simulink model "asbhl20_FDIRApp1"  (R2013a)
settings: Solver=FixedStepDiscrete  SolverMode=SingleTasking  StartTime=0.0  StopTime=10.0  FixedStep=1/60  RelTol=1e-3
PreLoadFcn:
  | load asbhl20GlobalChildrenData.mat
  | load asbhl20_FDIRAppData.mat
undefined symbols (not defined in the file): Tc, Tf
libraries: asbhl20screen x21, asbhl20_mode_logic x1
Description:
  | HL-20 actuators: fault detection, isolation, and recovery (FDIR) example module
settings Model: FPTRunName=Active  ExtModeAutoUpdateStatusClock=off  BufferReuse=off  Creator=The MathWorks Inc.
settings DataIOCC: LimitDataPoints=off  SaveOutput=off  SaveTime=off
settings OptimizationCC: BlockReduction=off  InlineParams=on  OptimizeBlockIOStorage=off  BufferReuse=off  ExpressionFolding=off  ExpressionDepthLimit=2147483647  LocalBlockOutputs=off  StateBitsets=on  DataBitsets=on  UseTempVars=on  InitFltsAndDblsToZero=on
settings DebuggingCC: SaveWithParameterizedLinksMsg=none  UnderspecifiedInitializationDetection=Simplified  MergeDetectMultiDrivingBlocksExec=error  MultiTaskCondExecSysMsg=none  FcnCallInpInsideContextMsg=EnableAllAsWarning  UniqueDataStoreMsg=error  StrictBusMsg=ErrorOnBusTreatedAsVector
settings HardwareCC: TargetHWDeviceType=32-bit Generic
settings ModelReferenceCC: UpdateModelReferenceTargets=AssumeUpToDate  CheckModelReferenceTargetMessage=none  ModelReferencePassRootInputsByReference=off
settings SFSimCC: SimParseCustomCode=off
settings RTWCC: ProcessScript=grt_make_rtw_hook  IncludeERTFirstTime=on
settings CodeAppCC: MaxIdLength=63
settings GRTTargetCC: TargetFcnLib=ansi_tfl_tmw.mat  CombineOutputUpdateFcns=off  GRTInterface=on

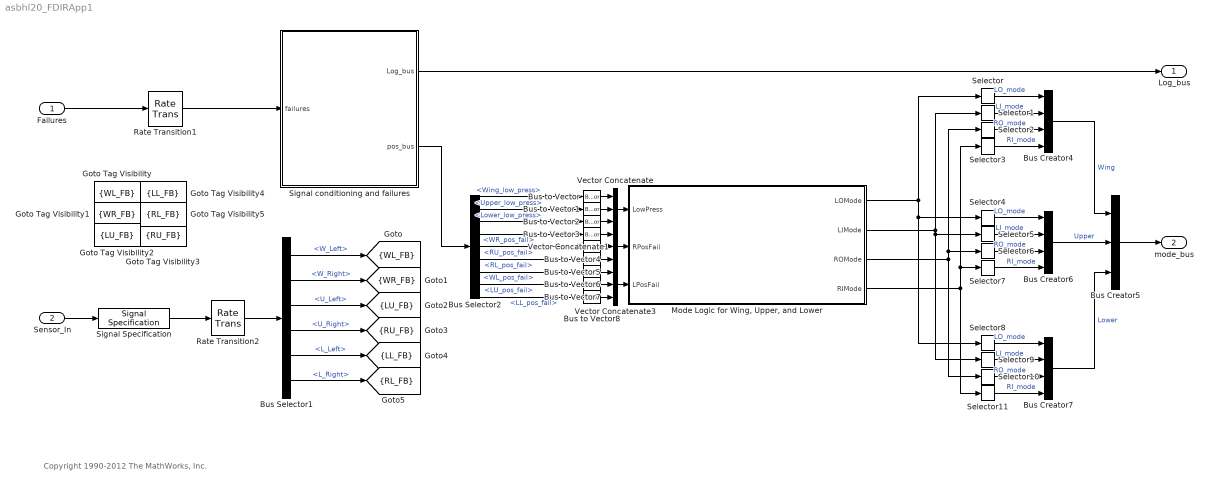
== system asbhl20_FDIRApp1 ==
  note: Copyright 1990-2012 The MathWorks, Inc.
  Failures : Inport  PortDimensions=21  SampleTime=Tc
  Sensor_In : Inport  Port=2  OutDataTypeStr=Bus: AirDataBus
  Bus Creator4 : BusCreator  OutDataTypeStr=Bus: ActuatorModeBus
  Bus Creator5 : BusCreator  Inputs=3  OutDataTypeStr=Bus: SurfaceModesBus
  Bus Creator6 : BusCreator  OutDataTypeStr=Bus: ActuatorModeBus
  Bus Creator7 : BusCreator  OutDataTypeStr=Bus: ActuatorModeBus
  Bus Selector1 : BusSelector  OutputSignals=W_Left,W_Right,U_Left,U_Right,L_Left,L_Right
  Bus Selector2 : BusSelector  OutputSignals=Wing_low_press,Upper_low_press,Lower_low_press,WR_pos_fail,RU_pos_fail,RL_pos_fail,WL_pos_fail,LU_pos_fail,LL_pos_fail
  Bus to Vector{,1..8} (9 alike) : BusToVector
  Goto Tag Visibility : GotoTagVisibility  GotoTag=WL_FB
  Goto Tag Visibility1 : GotoTagVisibility  GotoTag=WR_FB
  Goto Tag Visibility2 : GotoTagVisibility  GotoTag=LU_FB
  Goto Tag Visibility3 : GotoTagVisibility  GotoTag=RU_FB
  Goto Tag Visibility4 : GotoTagVisibility  GotoTag=LL_FB
  Goto Tag Visibility5 : GotoTagVisibility  GotoTag=RL_FB
  "Mode Logic for Wing, Upper, and Lower" : Subsystem  TreatAsAtomicUnit=on
  Rate Transition1 : RateTransition  OutPortSampleTime=Tf
  Rate Transition2 : RateTransition  OutPortSampleTime=Tf
  Selector{,1..3} (4 alike) : Selector  InputPortWidth=3  IndexOptions=Index vector (dialog)  Indices=1  OutputSizes=1
  Selector{8..11} (4 alike) : Selector  InputPortWidth=3  IndexOptions=Index vector (dialog)  Indices=3  OutputSizes=1
  Selector{4..7} (4 alike) : Selector  InputPortWidth=3  IndexOptions=Index vector (dialog)  Indices=2  OutputSizes=1
  Signal Specification : SignalSpecification  SampleTime=Tc
  Signal conditioning and failures : Subsystem
  Vector Concatenate : Concatenate  NumInputs=3
  Vector Concatenate1 : Concatenate  NumInputs=3
  Vector Concatenate3 : Concatenate  NumInputs=3
  Log_bus : Outport  OutDataTypeStr=Bus: SurfaceEventLogBus
  mode_bus : Outport  Port=2  OutDataTypeStr=Bus: SurfaceModesBus
  tag scope: LL_FB=scoped, LU_FB=scoped, RL_FB=scoped, RU_FB=scoped, WL_FB=scoped, WR_FB=scoped
  wires:
  Signal conditioning and failures/1(Log_bus) -> Log_bus/1
  Failures/1 -> Rate Transition1/1
  Signal conditioning and failures/2(pos_bus) -> Bus Selector2/1
  Sensor_In/1 -> Signal Specification/1
  Bus Selector1/1 -> [WL_FB]  "<W_Left>"
  Bus Selector1/2 -> [WR_FB]  "<W_Right>"
  Bus Selector1/3 -> [LU_FB]  "<U_Left>"
  Bus Selector1/4 -> [RU_FB]  "<U_Right>"
  Bus Selector1/5 -> [LL_FB]  "<L_Left>"
  Bus Selector1/6 -> [RL_FB]  "<L_Right>"
  Rate Transition1/1 -> Signal conditioning and failures/1(failures)
  Rate Transition2/1 -> Bus Selector1/1
  Signal Specification/1 -> Rate Transition2/1
  Bus Selector2/1 -> Bus to Vector/1  "<Wing_low_press>"
  Bus Selector2/2 -> Bus to Vector1/1  "<Upper_low_press>"
  Bus Selector2/3 -> Bus to Vector2/1  "<Lower_low_press>"
  Bus Selector2/4 -> Bus to Vector3/1  "<WR_pos_fail>"
  Bus Selector2/5 -> Bus to Vector4/1  "<RU_pos_fail>"
  Bus Selector2/6 -> Bus to Vector5/1  "<RL_pos_fail>"
  Bus Selector2/7 -> Bus to Vector6/1  "<WL_pos_fail>"
  Bus Selector2/8 -> Bus to Vector7/1  "<LU_pos_fail>"
  Bus Selector2/9 -> Bus to Vector8/1  "<LL_pos_fail>"
  Vector Concatenate/1 -> "Mode Logic for Wing, Upper, and Lower"/1(LowPress)
  Vector Concatenate1/1 -> "Mode Logic for Wing, Upper, and Lower"/2(RPosFail)
  Vector Concatenate3/1 -> "Mode Logic for Wing, Upper, and Lower"/3(LPosFail)
  Bus Creator4/1 -> Bus Creator5/1  "Wing"
  Bus Creator6/1 -> Bus Creator5/2  "Upper"
  Bus Creator7/1 -> Bus Creator5/3  "Lower"
  Selector/1 -> Bus Creator4/1  "LO_mode"
  Selector1/1 -> Bus Creator4/2  "LI_mode"
  Selector2/1 -> Bus Creator4/3  "RO_mode"
  Selector3/1 -> Bus Creator4/4  "RI_mode"
  Selector4/1 -> Bus Creator6/1  "LO_mode"
  Selector5/1 -> Bus Creator6/2  "LI_mode"
  Selector6/1 -> Bus Creator6/3  "RO_mode"
  Selector7/1 -> Bus Creator6/4  "RI_mode"
  Selector8/1 -> Bus Creator7/1  "LO_mode"
  Selector9/1 -> Bus Creator7/2  "LI_mode"
  Selector10/1 -> Bus Creator7/3  "RO_mode"
  Selector11/1 -> Bus Creator7/4  "RI_mode"
  "Mode Logic for Wing, Upper, and Lower"/1(LOMode) -> Selector/1, Selector4/1, Selector8/1
  "Mode Logic for Wing, Upper, and Lower"/2(LIMode) -> Selector5/1, Selector9/1, Selector1/1
  "Mode Logic for Wing, Upper, and Lower"/3(ROMode) -> Selector6/1, Selector2/1, Selector10/1
  "Mode Logic for Wing, Upper, and Lower"/4(RIMode) -> Selector7/1, Selector3/1, Selector11/1
  Bus Creator5/1 -> mode_bus/1
  Bus to Vector/1 -> Vector Concatenate/1
  Bus to Vector1/1 -> Vector Concatenate/2
  Bus to Vector2/1 -> Vector Concatenate/3
  Bus to Vector3/1 -> Vector Concatenate1/1
  Bus to Vector4/1 -> Vector Concatenate1/2
  Bus to Vector5/1 -> Vector Concatenate1/3
  Bus to Vector6/1 -> Vector Concatenate3/1
  Bus to Vector7/1 -> Vector Concatenate3/2
  Bus to Vector8/1 -> Vector Concatenate3/3

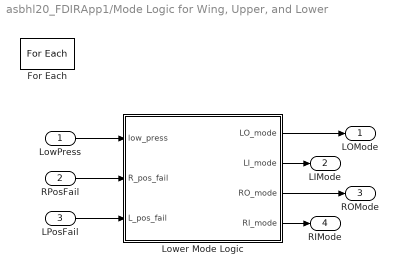
== system asbhl20_FDIRApp1/Mode Logic for Wing, Upper, and Lower ==
  LowPress : Inport  Partition=on  PartitionDimension=1  PartitionWidth=3
  RPosFail : Inport  Port=2  Partition=on  PartitionDimension=1  PartitionWidth=2
  LPosFail : Inport  Port=3  Partition=on  PartitionDimension=1  PartitionWidth=2
  For Each : ForEach  DisableCoverage=on  IndexMode=One-based
  Lower Mode Logic : Subsystem  BlockChoice=Mode Logic SS
      settings: TemplateBlock=asbhl20_mode_logic/Mode Logic  MemberBlocks=Mode Logic App,Mode Logic Chart,Mode Logic SS
  LOMode : Outport  ConcatenationDimension=1
  LIMode : Outport  Port=2  ConcatenationDimension=1
  ROMode : Outport  Port=3  ConcatenationDimension=1
  RIMode : Outport  Port=4  ConcatenationDimension=1
  wires:
  LPosFail/1 -> Lower Mode Logic/3(L_pos_fail)
  Lower Mode Logic/1(LO_mode) -> LOMode/1
  LowPress/1 -> Lower Mode Logic/1(low_press)
  RPosFail/1 -> Lower Mode Logic/2(R_pos_fail)
  Lower Mode Logic/2(LI_mode) -> LIMode/1
  Lower Mode Logic/3(RO_mode) -> ROMode/1
  Lower Mode Logic/4(RI_mode) -> RIMode/1

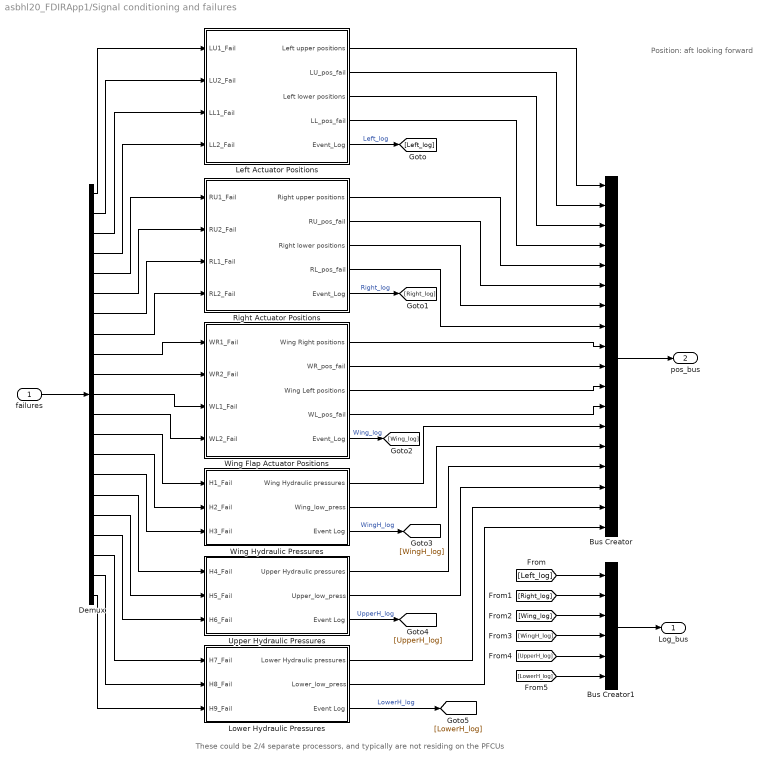
== system asbhl20_FDIRApp1/Signal conditioning and failures ==
  note: Position: aft looking forward
  note: These could be 2/4 separate processors, and typically are not residing on the PFCUs
  failures : Inport
  Bus Creator : BusCreator  Inputs=18
  Bus Creator1 : BusCreator  Inputs=6  OutDataTypeStr=Bus: SurfaceEventLogBus
  Demux : Demux  Outputs=21
  Left Actuator Positions : Subsystem
  Lower Hydraulic Pressures : Subsystem
  Right Actuator Positions : Subsystem
  Upper Hydraulic Pressures : Subsystem
  Wing Flap Actuator Positions : Subsystem
  Wing Hydraulic Pressures : Subsystem
  Log_bus : Outport  OutDataTypeStr=Bus: SurfaceEventLogBus
  pos_bus : Outport  Port=2
  wires:
  Bus Creator1/1 -> Log_bus/1
  [LowerH_log] -> Bus Creator1/6
  [UpperH_log] -> Bus Creator1/5
  [WingH_log] -> Bus Creator1/4
  [Wing_log] -> Bus Creator1/3
  [Right_log] -> Bus Creator1/2
  [Left_log] -> Bus Creator1/1
  Lower Hydraulic Pressures/3(Event Log) -> [LowerH_log]  "LowerH_log"
  Upper Hydraulic Pressures/3(Event Log) -> [UpperH_log]  "UpperH_log"
  Wing Hydraulic Pressures/3(Event Log) -> [WingH_log]  "WingH_log"
  Wing Flap Actuator Positions/5(Event_Log) -> [Wing_log]  "Wing_log"
  Right Actuator Positions/5(Event_Log) -> [Right_log]  "Right_log"
  Left Actuator Positions/5(Event_Log) -> [Left_log]  "Left_log"
  failures/1 -> Demux/1
  Demux/21 -> Lower Hydraulic Pressures/3(H9_Fail)
  Demux/20 -> Lower Hydraulic Pressures/2(H8_Fail)
  Demux/19 -> Lower Hydraulic Pressures/1(H7_Fail)
  Demux/18 -> Upper Hydraulic Pressures/3(H6_Fail)
  Demux/17 -> Upper Hydraulic Pressures/2(H5_Fail)
  Demux/16 -> Upper Hydraulic Pressures/1(H4_Fail)
  Demux/15 -> Wing Hydraulic Pressures/3(H3_Fail)
  Demux/14 -> Wing Hydraulic Pressures/2(H2_Fail)
  Demux/13 -> Wing Hydraulic Pressures/1(H1_Fail)
  Demux/12 -> Wing Flap Actuator Positions/4(WL2_Fail)
  Demux/11 -> Wing Flap Actuator Positions/3(WL1_Fail)
  Demux/10 -> Wing Flap Actuator Positions/2(WR2_Fail)
  Demux/9 -> Wing Flap Actuator Positions/1(WR1_Fail)
  Demux/8 -> Right Actuator Positions/4(RL2_Fail)
  Demux/7 -> Right Actuator Positions/3("RL1_Fail ")
  Demux/6 -> Right Actuator Positions/2(RU2_Fail)
  Demux/5 -> Right Actuator Positions/1(RU1_Fail)
  Demux/4 -> Left Actuator Positions/4("LL2_Fail ")
  Demux/3 -> Left Actuator Positions/3("LL1_Fail ")
  Demux/2 -> Left Actuator Positions/2("LU2_Fail ")
  Demux/1 -> Left Actuator Positions/1(LU1_Fail)
  Lower Hydraulic Pressures/2(Lower_low_press) -> Bus Creator/18
  Lower Hydraulic Pressures/1(Lower Hydraulic pressures) -> Bus Creator/17
  Upper Hydraulic Pressures/2(Upper_low_press) -> Bus Creator/16
  Upper Hydraulic Pressures/1(Upper Hydraulic pressures) -> Bus Creator/15
  Wing Hydraulic Pressures/2(Wing_low_press) -> Bus Creator/14
  Wing Hydraulic Pressures/1(Wing Hydraulic pressures) -> Bus Creator/13
  Wing Flap Actuator Positions/4(WL_pos_fail) -> Bus Creator/12
  Wing Flap Actuator Positions/3(Wing Left positions) -> Bus Creator/11
  Wing Flap Actuator Positions/2(WR_pos_fail) -> Bus Creator/10
  Wing Flap Actuator Positions/1(Wing Right positions) -> Bus Creator/9
  Right Actuator Positions/4(RL_pos_fail) -> Bus Creator/8
  Right Actuator Positions/3(Right lower positions) -> Bus Creator/7
  Right Actuator Positions/2(RU_pos_fail) -> Bus Creator/6
  Right Actuator Positions/1(Right upper positions) -> Bus Creator/5
  Left Actuator Positions/4(LL_pos_fail) -> Bus Creator/4
  Left Actuator Positions/3(Left lower positions) -> Bus Creator/3
  Left Actuator Positions/2(LU_pos_fail) -> Bus Creator/2
  Left Actuator Positions/1(Left upper positions) -> Bus Creator/1
  Bus Creator/1 -> pos_bus/1

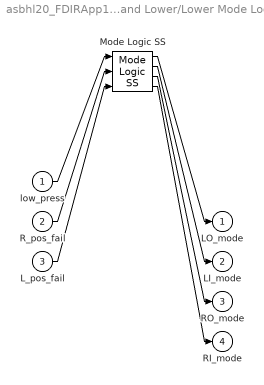
== system asbhl20_FDIRApp1/Mode Logic for Wing, Upper, and Lower/Lower Mode Logic ==
  low_press : Inport
  R_pos_fail : Inport  Port=2
  L_pos_fail : Inport  Port=3
  Mode Logic SS : asbhl20_mode_logic/Mode Logic SS
  LO_mode : Outport
  LI_mode : Outport  Port=2
  RO_mode : Outport  Port=3
  RI_mode : Outport  Port=4
  wires:
  low_press/1 -> Mode Logic SS/1
  R_pos_fail/1 -> Mode Logic SS/2
  L_pos_fail/1 -> Mode Logic SS/3
  Mode Logic SS/1 -> LO_mode/1
  Mode Logic SS/2 -> LI_mode/1
  Mode Logic SS/3 -> RO_mode/1
  Mode Logic SS/4 -> RI_mode/1

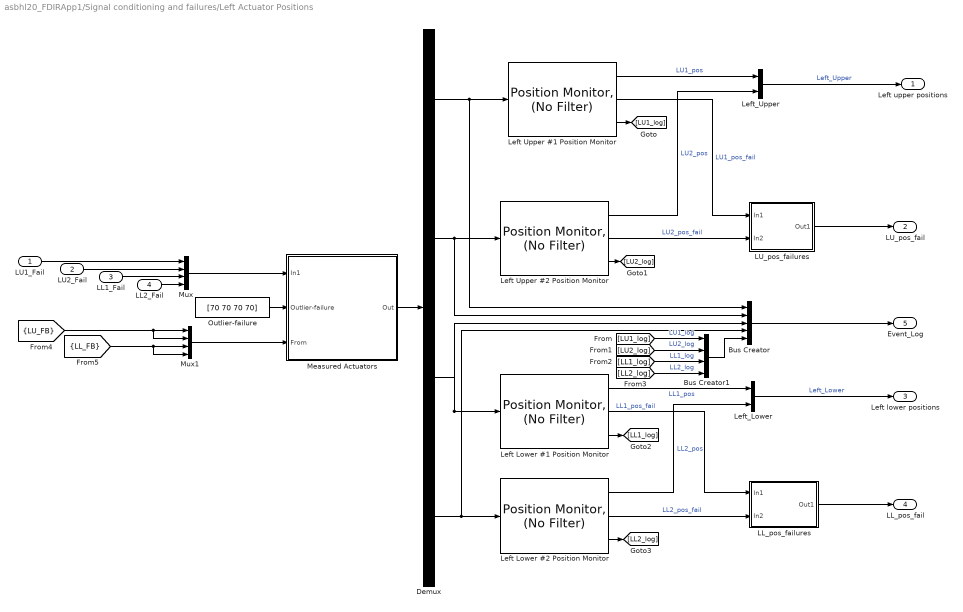
== system asbhl20_FDIRApp1/Signal conditioning and failures/Left Actuator Positions ==
  LU1_Fail : Inport
  "LU2_Fail " : Inport  Port=2
  "LL1_Fail " : Inport  Port=3
  "LL2_Fail " : Inport  Port=4
  Bus Creator : BusCreator  Inputs=5  OutDataTypeStr=Bus: LeftSurfaceEventBus
  Bus Creator1 : BusCreator  OutDataTypeStr=Bus: LeftSurfaceEventLogBus
  Demux : Demux  Outputs=[3 3 3 3]
  LL_pos_failures : Subsystem
  LU_pos_failures : Subsystem
  Left Lower #1 Position Monitor : asbhl20screen/Position Monitor, (No Filter)
  Left Lower #2 Position Monitor : asbhl20screen/Position Monitor, (No Filter)
  Left Upper #1 Position Monitor : asbhl20screen/Position Monitor, (No Filter)
  Left Upper #2 Position Monitor : asbhl20screen/Position Monitor, (No Filter)
  Left_Lower : BusCreator  Inputs=2
  Left_Upper : BusCreator  Inputs=2
  Measured Actuators : Subsystem  TreatAsAtomicUnit=on
  Mux : Mux
  Mux1 : Mux
  Outlier-failure : Constant  Value=[70 70 70 70]  SampleTime=Tf
  Left upper positions : Outport
  LU_pos_fail : Outport  Port=2
  Left lower positions : Outport  Port=3
  LL_pos_fail : Outport  Port=4
  Event_Log : Outport  Port=5  OutDataTypeStr=Bus: LeftSurfaceEventBus
  wires:
  [LL2_log] -> Bus Creator1/4  "LL2_log"
  [LL1_log] -> Bus Creator1/3  "LL1_log"
  [LU2_log] -> Bus Creator1/2  "LU2_log"
  [LU1_log] -> Bus Creator1/1  "LU1_log"
  Bus Creator1/1 -> Bus Creator/5
  "LL2_Fail "/1 -> Mux/4
  "LL1_Fail "/1 -> Mux/3
  "LU2_Fail "/1 -> Mux/2
  LU1_Fail/1 -> Mux/1
  Demux/2 -> Bus Creator/2, Left Upper #2 Position Monitor/1
  Demux/1 -> Bus Creator/1, Left Upper #1 Position Monitor/1
  Left Upper #1 Position Monitor/2 -> LU_pos_failures/1(In1)  "LU1_pos_fail"
  Left Lower #2 Position Monitor/3 -> [LL2_log]
  Left Lower #1 Position Monitor/3 -> [LL1_log]
  Left Upper #2 Position Monitor/3 -> [LU2_log]
  Left Upper #1 Position Monitor/3 -> [LU1_log]
  Bus Creator/1 -> Event_Log/1
  LL_pos_failures/1(Out1) -> LL_pos_fail/1
  Left_Lower/1 -> Left lower positions/1  "Left_Lower"
  LU_pos_failures/1(Out1) -> LU_pos_fail/1
  Left_Upper/1 -> Left upper positions/1  "Left_Upper"
  Left Lower #2 Position Monitor/2 -> LL_pos_failures/2(In2)  "LL2_pos_fail"
  Left Lower #2 Position Monitor/1 -> Left_Lower/2  "LL2_pos"
  Left Lower #1 Position Monitor/1 -> Left_Lower/1  "LL1_pos"
  Left Lower #1 Position Monitor/2 -> LL_pos_failures/1(In1)  "LL1_pos_fail"
  Left Upper #2 Position Monitor/2 -> LU_pos_failures/2(In2)  "LU2_pos_fail"
  Left Upper #2 Position Monitor/1 -> Left_Upper/2  "LU2_pos"
  Demux/4 -> Left Lower #2 Position Monitor/1, Bus Creator/4
  Demux/3 -> Bus Creator/3, Left Lower #1 Position Monitor/1
  Left Upper #1 Position Monitor/1 -> Left_Upper/1  "LU1_pos"
  Measured Actuators/1(Out) -> Demux/1
  Outlier-failure/1 -> Measured Actuators/2(Outlier-failure)
  Mux/1 -> Measured Actuators/1(In1)
  Mux1/1 -> Measured Actuators/3(From)
  [LU_FB] -> Mux1/1, Mux1/2
  [LL_FB] -> Mux1/3, Mux1/4

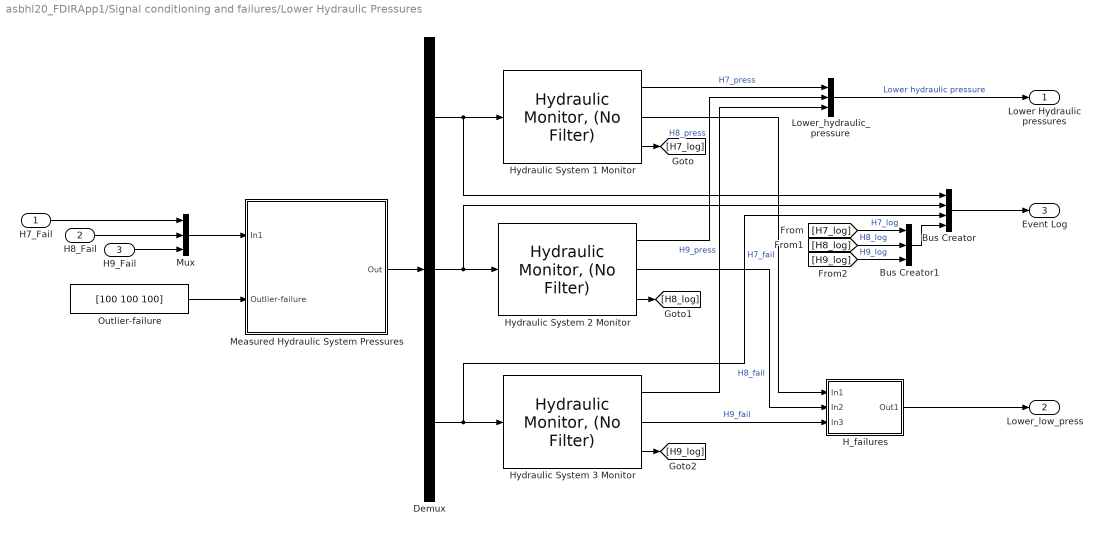
== system asbhl20_FDIRApp1/Signal conditioning and failures/Lower Hydraulic Pressures ==
  H7_Fail : Inport
  H8_Fail : Inport  Port=2
  H9_Fail : Inport  Port=3
  Bus Creator : BusCreator  OutDataTypeStr=Bus: LowerHydEventBus
  Bus Creator1 : BusCreator  Inputs=3  OutDataTypeStr=Bus: LowerHydEventLogBus
  Demux : Demux  Outputs=[3 3 3]
  H_failures : Subsystem
  Hydraulic System 1 Monitor : asbhl20screen/Hydraulic Monitor, (No Filter)
  Hydraulic System 2 Monitor : asbhl20screen/Hydraulic Monitor, (No Filter)
  Hydraulic System 3 Monitor : asbhl20screen/Hydraulic Monitor, (No Filter)
  Lower_hydraulic_pressure : BusCreator  Inputs=3
  Measured Hydraulic System Pressures : Subsystem  TreatAsAtomicUnit=on
  Mux : Mux  Inputs=3
  Outlier-failure : Constant  Value=[100 100 100]  SampleTime=Tf
  Lower Hydraulic pressures : Outport
  Lower_low_press : Outport  Port=2
  Event Log : Outport  Port=3  OutDataTypeStr=Bus: LowerHydEventBus
  wires:
  Bus Creator1/1 -> Bus Creator/4
  [H9_log] -> Bus Creator1/3  "H9_log"
  [H8_log] -> Bus Creator1/2  "H8_log"
  [H7_log] -> Bus Creator1/1  "H7_log"
  H8_Fail/1 -> Mux/2
  Hydraulic System 1 Monitor/3 -> [H7_log]
  Hydraulic System 2 Monitor/3 -> [H8_log]
  Hydraulic System 3 Monitor/3 -> [H9_log]
  Bus Creator/1 -> Event Log/1
  Demux/1 -> Bus Creator/1, Hydraulic System 1 Monitor/1
  Demux/2 -> Bus Creator/2, Hydraulic System 2 Monitor/1
  Hydraulic System 1 Monitor/1 -> Lower_hydraulic_pressure/1  "H7_press"
  Demux/3 -> Bus Creator/3, Hydraulic System 3 Monitor/1
  Hydraulic System 2 Monitor/1 -> Lower_hydraulic_pressure/2  "H8_press"
  Hydraulic System 1 Monitor/2 -> H_failures/1(In1)  "H7_fail"
  Hydraulic System 2 Monitor/2 -> H_failures/2(In2)  "H8_fail"
  Hydraulic System 3 Monitor/2 -> H_failures/3(In3)  "H9_fail"
  Hydraulic System 3 Monitor/1 -> Lower_hydraulic_pressure/3  "H9_press"
  H_failures/1(Out1) -> Lower_low_press/1
  H9_Fail/1 -> Mux/3
  H7_Fail/1 -> Mux/1
  Mux/1 -> Measured Hydraulic System Pressures/1(In1)
  Measured Hydraulic System Pressures/1(Out) -> Demux/1
  Outlier-failure/1 -> Measured Hydraulic System Pressures/2(Outlier-failure)
  Lower_hydraulic_pressure/1 -> Lower Hydraulic pressures/1  "Lower hydraulic pressure"

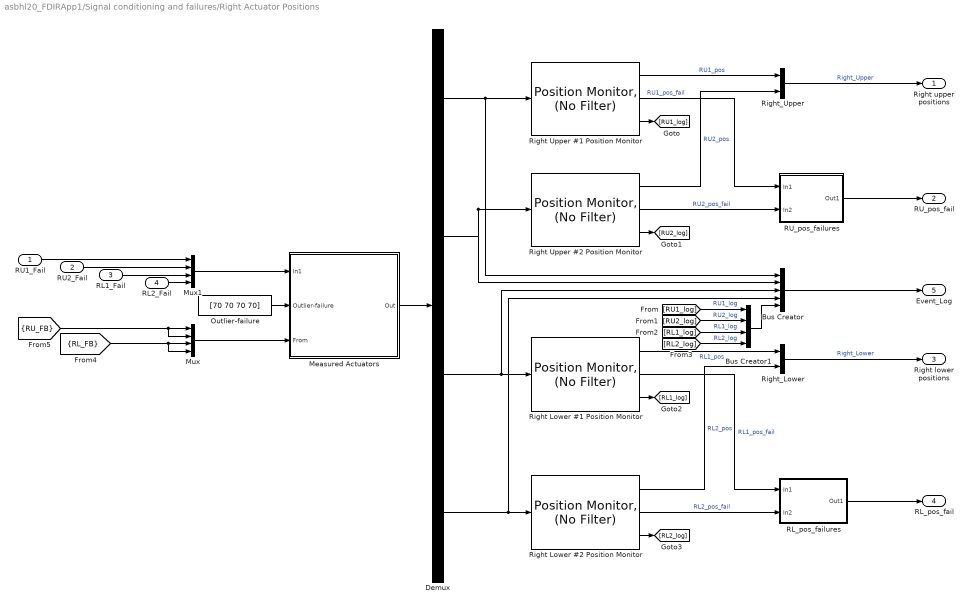
== system asbhl20_FDIRApp1/Signal conditioning and failures/Right Actuator Positions ==
  RU1_Fail : Inport
  RU2_Fail : Inport  Port=2
  "RL1_Fail " : Inport  Port=3
  RL2_Fail : Inport  Port=4
  Bus Creator : BusCreator  Inputs=5  OutDataTypeStr=Bus: RightSurfaceEventBus
  Bus Creator1 : BusCreator  OutDataTypeStr=Bus: RightSurfaceEventLogBus
  Demux : Demux  Outputs=[3 3 3 3]
  Measured Actuators : Subsystem  TreatAsAtomicUnit=on
  Mux : Mux
  Mux1 : Mux
  Outlier-failure : Constant  Value=[70 70 70 70]  SampleTime=Tf
  RL_pos_failures : Subsystem
  RU_pos_failures : Subsystem
  Right Lower #1 Position Monitor : asbhl20screen/Position Monitor, (No Filter)
  Right Lower #2 Position Monitor : asbhl20screen/Position Monitor, (No Filter)
  Right Upper #1 Position Monitor : asbhl20screen/Position Monitor, (No Filter)
  Right Upper #2 Position Monitor : asbhl20screen/Position Monitor, (No Filter)
  Right_Lower : BusCreator  Inputs=2
  Right_Upper : BusCreator  Inputs=2
  Right upper positions : Outport
  RU_pos_fail : Outport  Port=2
  Right lower positions : Outport  Port=3
  RL_pos_fail : Outport  Port=4
  Event_Log : Outport  Port=5  OutDataTypeStr=Bus: RightSurfaceEventBus
  wires:
  [RL2_log] -> Bus Creator1/4  "RL2_log"
  [RL1_log] -> Bus Creator1/3  "RL1_log"
  [RU2_log] -> Bus Creator1/2  "RU2_log"
  [RU1_log] -> Bus Creator1/1  "RU1_log"
  Bus Creator1/1 -> Bus Creator/5
  RL2_Fail/1 -> Mux1/4
  "RL1_Fail "/1 -> Mux1/3
  RU2_Fail/1 -> Mux1/2
  RU1_Fail/1 -> Mux1/1
  Right Upper #1 Position Monitor/1 -> Right_Upper/1  "RU1_pos"
  Demux/3 -> Right Lower #1 Position Monitor/1, Bus Creator/3
  Demux/4 -> Bus Creator/4, Right Lower #2 Position Monitor/1
  Right Upper #2 Position Monitor/1 -> Right_Upper/2  "RU2_pos"
  Right Upper #2 Position Monitor/2 -> RU_pos_failures/2(In2)  "RU2_pos_fail"
  Right Lower #1 Position Monitor/2 -> RL_pos_failures/1(In1)  "RL1_pos_fail"
  Right Lower #1 Position Monitor/1 -> Right_Lower/1  "RL1_pos"
  Right Lower #2 Position Monitor/1 -> Right_Lower/2  "RL2_pos"
  Right Lower #2 Position Monitor/2 -> RL_pos_failures/2(In2)  "RL2_pos_fail"
  Right_Upper/1 -> Right upper positions/1  "Right_Upper"
  RU_pos_failures/1(Out1) -> RU_pos_fail/1
  Right_Lower/1 -> Right lower positions/1  "Right_Lower"
  RL_pos_failures/1(Out1) -> RL_pos_fail/1
  Bus Creator/1 -> Event_Log/1
  Right Upper #1 Position Monitor/3 -> [RU1_log]
  Right Upper #2 Position Monitor/3 -> [RU2_log]
  Right Lower #1 Position Monitor/3 -> [RL1_log]
  Right Lower #2 Position Monitor/3 -> [RL2_log]
  Right Upper #1 Position Monitor/2 -> RU_pos_failures/1(In1)  "RU1_pos_fail"
  Demux/1 -> Right Upper #1 Position Monitor/1, Bus Creator/1
  Demux/2 -> Right Upper #2 Position Monitor/1, Bus Creator/2
  Measured Actuators/1(Out) -> Demux/1
  Outlier-failure/1 -> Measured Actuators/2(Outlier-failure)
  Mux1/1 -> Measured Actuators/1(In1)
  Mux/1 -> Measured Actuators/3(From)
  [RU_FB] -> Mux/1, Mux/2
  [RL_FB] -> Mux/3, Mux/4

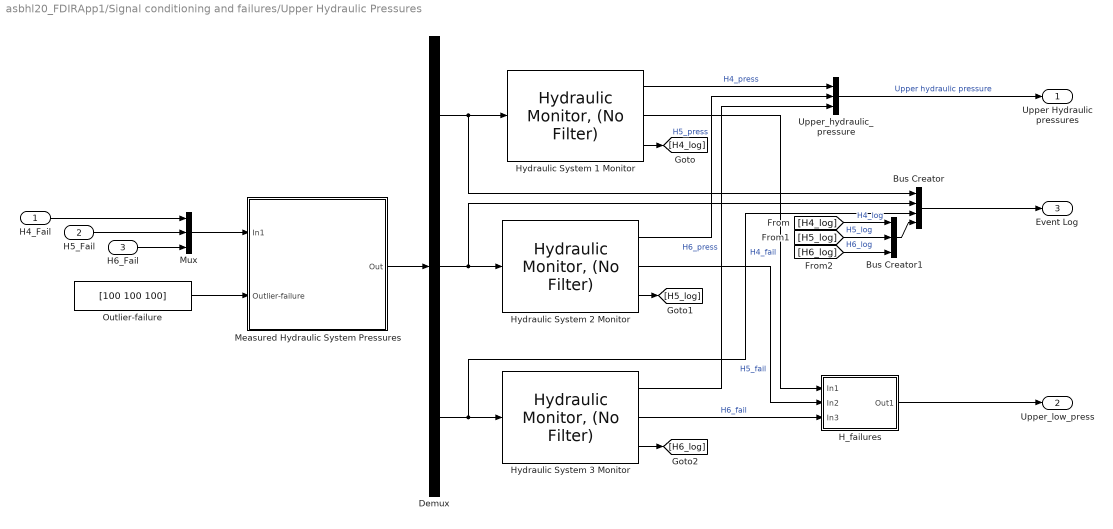
== system asbhl20_FDIRApp1/Signal conditioning and failures/Upper Hydraulic Pressures ==
  H4_Fail : Inport
  H5_Fail : Inport  Port=2
  H6_Fail : Inport  Port=3
  Bus Creator : BusCreator  OutDataTypeStr=Bus: UpperHydEventBus
  Bus Creator1 : BusCreator  Inputs=3  OutDataTypeStr=Bus: UpperHydEventLogBus
  Demux : Demux  Outputs=[3 3 3]
  H_failures : Subsystem
  Hydraulic System 1 Monitor : asbhl20screen/Hydraulic Monitor, (No Filter)
  Hydraulic System 2 Monitor : asbhl20screen/Hydraulic Monitor, (No Filter)
  Hydraulic System 3 Monitor : asbhl20screen/Hydraulic Monitor, (No Filter)
  Measured Hydraulic System Pressures : Subsystem  TreatAsAtomicUnit=on
  Mux : Mux  Inputs=3
  Outlier-failure : Constant  Value=[100 100 100]  SampleTime=Tf
  Upper_hydraulic_pressure : BusCreator  Inputs=3
  Upper Hydraulic pressures : Outport
  Upper_low_press : Outport  Port=2
  Event Log : Outport  Port=3  OutDataTypeStr=Bus: UpperHydEventBus
  wires:
  Bus Creator1/1 -> Bus Creator/4
  [H6_log] -> Bus Creator1/3  "H6_log"
  [H5_log] -> Bus Creator1/2  "H5_log"
  [H4_log] -> Bus Creator1/1  "H4_log"
  H6_Fail/1 -> Mux/3
  H5_Fail/1 -> Mux/2
  H4_Fail/1 -> Mux/1
  H_failures/1(Out1) -> Upper_low_press/1
  Upper_hydraulic_pressure/1 -> Upper Hydraulic pressures/1  "Upper hydraulic pressure"
  Hydraulic System 3 Monitor/1 -> Upper_hydraulic_pressure/3  "H6_press"
  Hydraulic System 3 Monitor/2 -> H_failures/3(In3)  "H6_fail"
  Hydraulic System 2 Monitor/2 -> H_failures/2(In2)  "H5_fail"
  Hydraulic System 1 Monitor/2 -> H_failures/1(In1)  "H4_fail"
  Hydraulic System 2 Monitor/1 -> Upper_hydraulic_pressure/2  "H5_press"
  Demux/3 -> Hydraulic System 3 Monitor/1, Bus Creator/3
  Hydraulic System 1 Monitor/1 -> Upper_hydraulic_pressure/1  "H4_press"
  Demux/2 -> Hydraulic System 2 Monitor/1, Bus Creator/2
  Demux/1 -> Hydraulic System 1 Monitor/1, Bus Creator/1
  Bus Creator/1 -> Event Log/1
  Hydraulic System 3 Monitor/3 -> [H6_log]
  Hydraulic System 2 Monitor/3 -> [H5_log]
  Hydraulic System 1 Monitor/3 -> [H4_log]
  Mux/1 -> Measured Hydraulic System Pressures/1(In1)
  Measured Hydraulic System Pressures/1(Out) -> Demux/1
  Outlier-failure/1 -> Measured Hydraulic System Pressures/2(Outlier-failure)

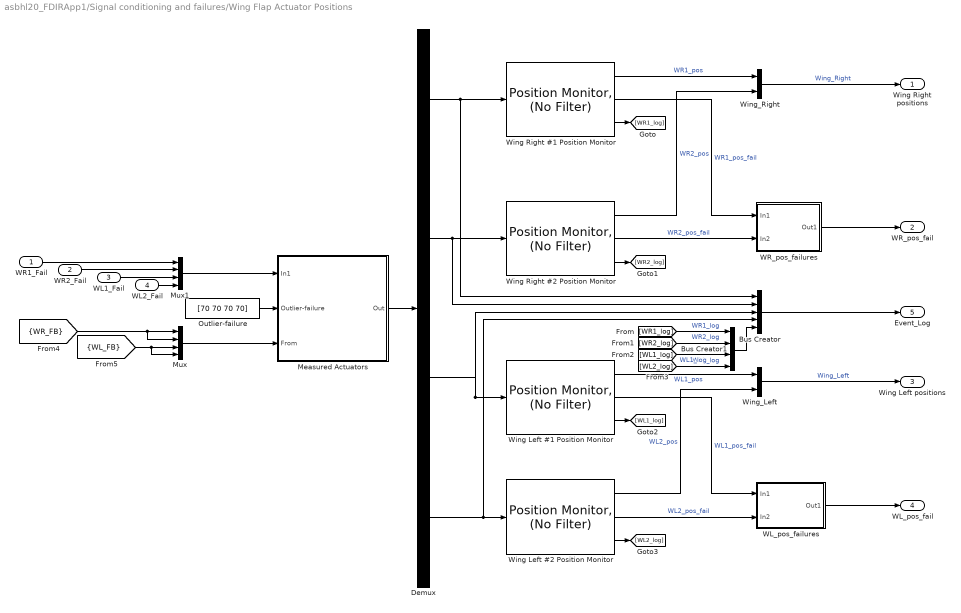
== system asbhl20_FDIRApp1/Signal conditioning and failures/Wing Flap Actuator Positions ==
  WR1_Fail : Inport
  WR2_Fail : Inport  Port=2
  WL1_Fail : Inport  Port=3
  WL2_Fail : Inport  Port=4
  Bus Creator : BusCreator  Inputs=5  OutDataTypeStr=Bus: WingSurfaceEventBus
  Bus Creator1 : BusCreator  OutDataTypeStr=Bus: WingSurfaceEventLogBus
  Demux : Demux  Outputs=[3 3 3 3]
  Measured Actuators : Subsystem  TreatAsAtomicUnit=on
  Mux : Mux
  Mux1 : Mux
  Outlier-failure : Constant  Value=[70 70 70 70]  SampleTime=Tf
  WL_pos_failures : Subsystem
  WR_pos_failures : Subsystem
  Wing Left #1 Position Monitor : asbhl20screen/Position Monitor, (No Filter)
  Wing Left #2 Position Monitor : asbhl20screen/Position Monitor, (No Filter)
  Wing Right #1 Position Monitor : asbhl20screen/Position Monitor, (No Filter)
  Wing Right #2 Position Monitor : asbhl20screen/Position Monitor, (No Filter)
  Wing_Left : BusCreator  Inputs=2
  Wing_Right : BusCreator  Inputs=2
  Wing Right positions : Outport
  WR_pos_fail : Outport  Port=2
  Wing Left positions : Outport  Port=3
  WL_pos_fail : Outport  Port=4
  Event_Log : Outport  Port=5  OutDataTypeStr=Bus: WingSurfaceEventBus
  wires:
  [WL2_log] -> Bus Creator1/4  "WL2_log"
  [WL1_log] -> Bus Creator1/3  "WL1_log"
  [WR2_log] -> Bus Creator1/2  "WR2_log"
  [WR1_log] -> Bus Creator1/1  "WR1_log"
  Bus Creator1/1 -> Bus Creator/5
  WL2_Fail/1 -> Mux1/4
  WL1_Fail/1 -> Mux1/3
  WR2_Fail/1 -> Mux1/2
  WR1_Fail/1 -> Mux1/1
  Demux/2 -> Bus Creator/2, Wing Right #2 Position Monitor/1
  Demux/1 -> Bus Creator/1, Wing Right #1 Position Monitor/1
  Wing Right #1 Position Monitor/2 -> WR_pos_failures/1(In1)  "WR1_pos_fail"
  Wing Left #2 Position Monitor/3 -> [WL2_log]
  Wing Left #1 Position Monitor/3 -> [WL1_log]
  Wing Right #2 Position Monitor/3 -> [WR2_log]
  Wing Right #1 Position Monitor/3 -> [WR1_log]
  Bus Creator/1 -> Event_Log/1
  WL_pos_failures/1(Out1) -> WL_pos_fail/1
  Wing_Left/1 -> Wing Left positions/1  "Wing_Left"
  WR_pos_failures/1(Out1) -> WR_pos_fail/1
  Wing_Right/1 -> Wing Right positions/1  "Wing_Right"
  Wing Left #2 Position Monitor/2 -> WL_pos_failures/2(In2)  "WL2_pos_fail"
  Wing Left #2 Position Monitor/1 -> Wing_Left/2  "WL2_pos"
  Wing Left #1 Position Monitor/1 -> Wing_Left/1  "WL1_pos"
  Wing Left #1 Position Monitor/2 -> WL_pos_failures/1(In1)  "WL1_pos_fail"
  Wing Right #2 Position Monitor/2 -> WR_pos_failures/2(In2)  "WR2_pos_fail"
  Wing Right #2 Position Monitor/1 -> Wing_Right/2  "WR2_pos"
  Demux/4 -> Wing Left #2 Position Monitor/1, Bus Creator/4
  Demux/3 -> Bus Creator/3, Wing Left #1 Position Monitor/1
  Wing Right #1 Position Monitor/1 -> Wing_Right/1  "WR1_pos"
  Measured Actuators/1(Out) -> Demux/1
  Outlier-failure/1 -> Measured Actuators/2(Outlier-failure)
  Mux1/1 -> Measured Actuators/1(In1)
  Mux/1 -> Measured Actuators/3(From)
  [WR_FB] -> Mux/1, Mux/2
  [WL_FB] -> Mux/3, Mux/4

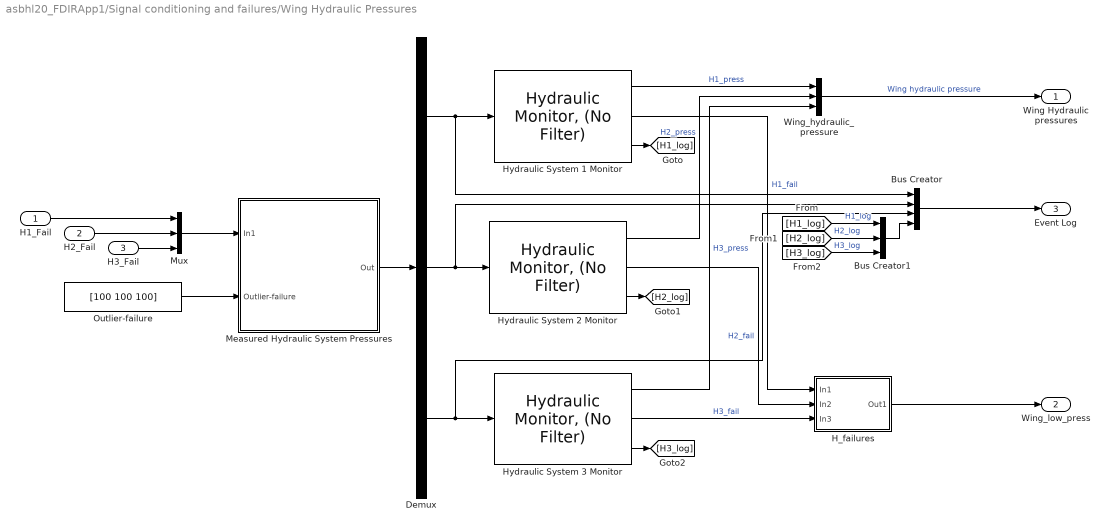
== system asbhl20_FDIRApp1/Signal conditioning and failures/Wing Hydraulic Pressures ==
  H1_Fail : Inport
  H2_Fail : Inport  Port=2
  H3_Fail : Inport  Port=3
  Bus Creator : BusCreator  OutDataTypeStr=Bus: WingHydEventBus
  Bus Creator1 : BusCreator  Inputs=3  OutDataTypeStr=Bus: WingHydEventLogBus
  Demux : Demux  Outputs=[3 3 3]
  H_failures : Subsystem
  Hydraulic System 1 Monitor : asbhl20screen/Hydraulic Monitor, (No Filter)
  Hydraulic System 2 Monitor : asbhl20screen/Hydraulic Monitor, (No Filter)
  Hydraulic System 3 Monitor : asbhl20screen/Hydraulic Monitor, (No Filter)
  Measured Hydraulic System Pressures : Subsystem  TreatAsAtomicUnit=on
  Mux : Mux  Inputs=3
  Outlier-failure : Constant  Value=[100 100 100]  SampleTime=Tf
  Wing_hydraulic_pressure : BusCreator  Inputs=3
  Wing Hydraulic pressures : Outport
  Wing_low_press : Outport  Port=2
  Event Log : Outport  Port=3  OutDataTypeStr=Bus: WingHydEventBus
  wires:
  [H3_log] -> Bus Creator1/3  "H3_log"
  [H2_log] -> Bus Creator1/2  "H2_log"
  [H1_log] -> Bus Creator1/1  "H1_log"
  Bus Creator1/1 -> Bus Creator/4
  H3_Fail/1 -> Mux/3
  H2_Fail/1 -> Mux/2
  H1_Fail/1 -> Mux/1
  Hydraulic System 1 Monitor/3 -> [H1_log]
  Hydraulic System 2 Monitor/3 -> [H2_log]
  Hydraulic System 3 Monitor/3 -> [H3_log]
  Bus Creator/1 -> Event Log/1
  Demux/1 -> Bus Creator/1, Hydraulic System 1 Monitor/1
  Demux/2 -> Bus Creator/2, Hydraulic System 2 Monitor/1
  Hydraulic System 1 Monitor/1 -> Wing_hydraulic_pressure/1  "H1_press"
  Demux/3 -> Bus Creator/3, Hydraulic System 3 Monitor/1
  Hydraulic System 2 Monitor/1 -> Wing_hydraulic_pressure/2  "H2_press"
  Hydraulic System 1 Monitor/2 -> H_failures/1(In1)  "H1_fail"
  Hydraulic System 2 Monitor/2 -> H_failures/2(In2)  "H2_fail"
  Hydraulic System 3 Monitor/2 -> H_failures/3(In3)  "H3_fail"
  Hydraulic System 3 Monitor/1 -> Wing_hydraulic_pressure/3  "H3_press"
  H_failures/1(Out1) -> Wing_low_press/1
  Mux/1 -> Measured Hydraulic System Pressures/1(In1)
  Measured Hydraulic System Pressures/1(Out) -> Demux/1
  Outlier-failure/1 -> Measured Hydraulic System Pressures/2(Outlier-failure)
  Wing_hydraulic_pressure/1 -> Wing Hydraulic pressures/1  "Wing hydraulic pressure"

== system asbhl20_FDIRApp1/Signal conditioning and failures/Left Actuator Positions/LL_pos_failures ==
  In1 : Inport
  In2 : Inport  Port=2
  LL_pos_fail : BusCreator  Inputs=2
  Out1 : Outport
  wires:
  In2/1 -> LL_pos_fail/2
  LL_pos_fail/1 -> Out1/1  "LL_pos_fail"
  In1/1 -> LL_pos_fail/1

== system asbhl20_FDIRApp1/Signal conditioning and failures/Left Actuator Positions/LU_pos_failures ==
  In1 : Inport
  In2 : Inport  Port=2
  LU_pos_fail : BusCreator  Inputs=2
  Out1 : Outport
  wires:
  In2/1 -> LU_pos_fail/2
  LU_pos_fail/1 -> Out1/1  "LU_pos_fail"
  In1/1 -> LU_pos_fail/1

== system asbhl20_FDIRApp1/Signal conditioning and failures/Left Actuator Positions/Measured Actuators ==
  In1 : Inport  Partition=on  PartitionDimension=1  PartitionWidth=1
  Outlier-failure : Inport  Port=2  Partition=on  PartitionDimension=1  PartitionWidth=1
  From : Inport  Port=3  Partition=on  PartitionDimension=1  PartitionWidth=1
  For Each : ForEach  DisableCoverage=on  IndexMode=One-based
  Measured Actuator : Subsystem
  Out : Outport  ConcatenationDimension=1
  wires:
  Outlier-failure/1 -> Measured Actuator/2(Outlier-failure)
  In1/1 -> Measured Actuator/1(In3)
  Measured Actuator/1(Out) -> Out/1
  From/1 -> Measured Actuator/3(From)

== system asbhl20_FDIRApp1/Signal conditioning and failures/Lower Hydraulic Pressures/H_failures ==
  In1 : Inport
  In2 : Inport  Port=2
  In3 : Inport  Port=3
  Lower_low_pressure : BusCreator  Inputs=3
  Out1 : Outport
  wires:
  In3/1 -> Lower_low_pressure/3
  In2/1 -> Lower_low_pressure/2
  In1/1 -> Lower_low_pressure/1
  Lower_low_pressure/1 -> Out1/1  "Lower_low_press"

== system asbhl20_FDIRApp1/Signal conditioning and failures/Lower Hydraulic Pressures/Measured Hydraulic System Pressures ==
  In1 : Inport  Partition=on  PartitionDimension=1  PartitionWidth=1
  Outlier-failure : Inport  Port=2  Partition=on  PartitionDimension=1  PartitionWidth=1
  For Each : ForEach  DisableCoverage=on  IndexMode=One-based
  Measured Hydraulic system 1 pressures : Subsystem
  Out : Outport  ConcatenationDimension=1
  wires:
  Outlier-failure/1 -> Measured Hydraulic system 1 pressures/2(Outlier-failure)
  In1/1 -> Measured Hydraulic system 1 pressures/1(In3)
  Measured Hydraulic system 1 pressures/1(Out) -> Out/1

== system asbhl20_FDIRApp1/Signal conditioning and failures/Right Actuator Positions/Measured Actuators ==
  In1 : Inport  Partition=on  PartitionDimension=1  PartitionWidth=1
  Outlier-failure : Inport  Port=2  Partition=on  PartitionDimension=1  PartitionWidth=1
  From : Inport  Port=3  Partition=on  PartitionDimension=1  PartitionWidth=1
  For Each : ForEach  DisableCoverage=on  IndexMode=One-based
  Measured Actuator : Subsystem
  Out : Outport  ConcatenationDimension=1
  wires:
  Outlier-failure/1 -> Measured Actuator/2(Outlier-failure)
  In1/1 -> Measured Actuator/1(In3)
  Measured Actuator/1(Out) -> Out/1
  From/1 -> Measured Actuator/3(From)

== system asbhl20_FDIRApp1/Signal conditioning and failures/Right Actuator Positions/RL_pos_failures ==
  In1 : Inport
  In2 : Inport  Port=2
  RL_pos_fail : BusCreator  Inputs=2
  Out1 : Outport
  wires:
  In1/1 -> RL_pos_fail/1
  RL_pos_fail/1 -> Out1/1  "RL_pos_fail"
  In2/1 -> RL_pos_fail/2

== system asbhl20_FDIRApp1/Signal conditioning and failures/Right Actuator Positions/RU_pos_failures ==
  In1 : Inport
  In2 : Inport  Port=2
  RU_pos_fail : BusCreator  Inputs=2
  Out1 : Outport
  wires:
  In1/1 -> RU_pos_fail/1
  RU_pos_fail/1 -> Out1/1  "RU_pos_fail"
  In2/1 -> RU_pos_fail/2

== system asbhl20_FDIRApp1/Signal conditioning and failures/Upper Hydraulic Pressures/H_failures ==
  In1 : Inport
  In2 : Inport  Port=2
  In3 : Inport  Port=3
  Upper_low_pressure : BusCreator  Inputs=3
  Out1 : Outport
  wires:
  Upper_low_pressure/1 -> Out1/1  "Upper_low_press"
  In1/1 -> Upper_low_pressure/1
  In2/1 -> Upper_low_pressure/2
  In3/1 -> Upper_low_pressure/3

== system asbhl20_FDIRApp1/Signal conditioning and failures/Upper Hydraulic Pressures/Measured Hydraulic System Pressures ==
  In1 : Inport  Partition=on  PartitionDimension=1  PartitionWidth=1
  Outlier-failure : Inport  Port=2  Partition=on  PartitionDimension=1  PartitionWidth=1
  For Each : ForEach  DisableCoverage=on  IndexMode=One-based
  Measured Hydraulic system 1 pressures : Subsystem
  Out : Outport  ConcatenationDimension=1
  wires:
  Measured Hydraulic system 1 pressures/1(Out) -> Out/1
  In1/1 -> Measured Hydraulic system 1 pressures/1(In3)
  Outlier-failure/1 -> Measured Hydraulic system 1 pressures/2(Outlier-failure)

== system asbhl20_FDIRApp1/Signal conditioning and failures/Wing Flap Actuator Positions/Measured Actuators ==
  In1 : Inport  Partition=on  PartitionDimension=1  PartitionWidth=1
  Outlier-failure : Inport  Port=2  Partition=on  PartitionDimension=1  PartitionWidth=1
  From : Inport  Port=3  Partition=on  PartitionDimension=1  PartitionWidth=1
  For Each : ForEach  DisableCoverage=on  IndexMode=One-based
  Measured Actuator : Subsystem
  Out : Outport  ConcatenationDimension=1
  wires:
  From/1 -> Measured Actuator/3(From)
  Measured Actuator/1(Out) -> Out/1
  In1/1 -> Measured Actuator/1(In3)
  Outlier-failure/1 -> Measured Actuator/2(Outlier-failure)

== system asbhl20_FDIRApp1/Signal conditioning and failures/Wing Flap Actuator Positions/WL_pos_failures ==
  In1 : Inport
  In2 : Inport  Port=2
  WL_pos_fail : BusCreator  Inputs=2
  Out1 : Outport
  wires:
  In2/1 -> WL_pos_fail/2
  WL_pos_fail/1 -> Out1/1  "WL_pos_fail"
  In1/1 -> WL_pos_fail/1

== system asbhl20_FDIRApp1/Signal conditioning and failures/Wing Flap Actuator Positions/WR_pos_failures ==
  In1 : Inport
  In2 : Inport  Port=2
  WR_pos_fail : BusCreator  Inputs=2
  Out1 : Outport
  wires:
  In2/1 -> WR_pos_fail/2
  WR_pos_fail/1 -> Out1/1  "WR_pos_fail"
  In1/1 -> WR_pos_fail/1

== system asbhl20_FDIRApp1/Signal conditioning and failures/Wing Hydraulic Pressures/H_failures ==
  In1 : Inport
  In2 : Inport  Port=2
  In3 : Inport  Port=3
  Wing_low_press : BusCreator  Inputs=3
  Out1 : Outport
  wires:
  In3/1 -> Wing_low_press/3
  In2/1 -> Wing_low_press/2
  In1/1 -> Wing_low_press/1
  Wing_low_press/1 -> Out1/1  "Wing_low_press"

== system asbhl20_FDIRApp1/Signal conditioning and failures/Wing Hydraulic Pressures/Measured Hydraulic System Pressures ==
  In1 : Inport  Partition=on  PartitionDimension=1  PartitionWidth=1
  Outlier-failure : Inport  Port=2  Partition=on  PartitionDimension=1  PartitionWidth=1
  For Each : ForEach  DisableCoverage=on  IndexMode=One-based
  Measured Hydraulic system 1 pressures : Subsystem
  Out : Outport  ConcatenationDimension=1
  wires:
  Measured Hydraulic system 1 pressures/1(Out) -> Out/1
  In1/1 -> Measured Hydraulic system 1 pressures/1(In3)
  Outlier-failure/1 -> Measured Hydraulic system 1 pressures/2(Outlier-failure)

== system asbhl20_FDIRApp1/Signal conditioning and failures/Left Actuator Positions/Measured Actuators/Measured Actuator ==
  In3 : Inport
  Outlier-failure : Inport  Port=2
  From : Inport  Port=3
  Gain : Gain  Gain=[1 1 1]
  Switch : Switch  Criteria=u2 ~= 0  SaturateOnIntegerOverflow=on
  Out : Outport
  wires:
  From/1 -> Switch/3
  In3/1 -> Switch/2
  Outlier-failure/1 -> Switch/1
  Gain/1 -> Out/1
  Switch/1 -> Gain/1

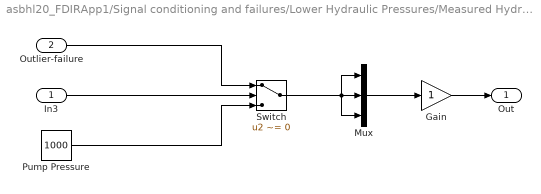
== system asbhl20_FDIRApp1/Signal conditioning and failures/Lower Hydraulic Pressures/Measured Hydraulic System Pressures/Measured Hydraulic system 1 pressures ==
  In3 : Inport
  Outlier-failure : Inport  Port=2
  Gain : Gain
  Mux : Mux  Inputs=3
  Pump Pressure : Constant  Value=1000
  Switch : Switch  Criteria=u2 ~= 0  SaturateOnIntegerOverflow=on
  Out : Outport
  wires:
  Pump Pressure/1 -> Switch/3
  In3/1 -> Switch/2
  Switch/1 -> Mux/2, Mux/1, Mux/3
  Mux/1 -> Gain/1
  Outlier-failure/1 -> Switch/1
  Gain/1 -> Out/1

== system asbhl20_FDIRApp1/Signal conditioning and failures/Right Actuator Positions/Measured Actuators/Measured Actuator ==
  In3 : Inport
  Outlier-failure : Inport  Port=2
  From : Inport  Port=3
  Gain : Gain  Gain=[1 1 1]
  Switch : Switch  Criteria=u2 ~= 0  SaturateOnIntegerOverflow=on
  Out : Outport
  wires:
  From/1 -> Switch/3
  In3/1 -> Switch/2
  Outlier-failure/1 -> Switch/1
  Gain/1 -> Out/1
  Switch/1 -> Gain/1

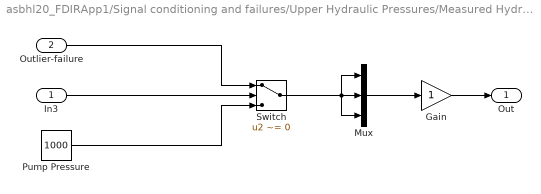
== system asbhl20_FDIRApp1/Signal conditioning and failures/Upper Hydraulic Pressures/Measured Hydraulic System Pressures/Measured Hydraulic system 1 pressures ==
  In3 : Inport
  Outlier-failure : Inport  Port=2
  Gain : Gain
  Mux : Mux  Inputs=3
  Pump Pressure : Constant  Value=1000
  Switch : Switch  Criteria=u2 ~= 0  SaturateOnIntegerOverflow=on
  Out : Outport
  wires:
  Gain/1 -> Out/1
  Outlier-failure/1 -> Switch/1
  Mux/1 -> Gain/1
  Switch/1 -> Mux/3, Mux/1, Mux/2
  In3/1 -> Switch/2
  Pump Pressure/1 -> Switch/3

== system asbhl20_FDIRApp1/Signal conditioning and failures/Wing Flap Actuator Positions/Measured Actuators/Measured Actuator ==
  In3 : Inport
  Outlier-failure : Inport  Port=2
  From : Inport  Port=3
  Gain : Gain  Gain=[1 1 1]
  Switch : Switch  Criteria=u2 ~= 0  SaturateOnIntegerOverflow=on
  Out : Outport
  wires:
  Switch/1 -> Gain/1
  Gain/1 -> Out/1
  Outlier-failure/1 -> Switch/1
  In3/1 -> Switch/2
  From/1 -> Switch/3

== system asbhl20_FDIRApp1/Signal conditioning and failures/Wing Hydraulic Pressures/Measured Hydraulic System Pressures/Measured Hydraulic system 1 pressures ==
  In3 : Inport
  Outlier-failure : Inport  Port=2
  Gain : Gain
  Mux : Mux  Inputs=3
  Pump Pressure : Constant  Value=1000
  Switch : Switch  Criteria=u2 ~= 0  SaturateOnIntegerOverflow=on
  Out : Outport
  wires:
  Gain/1 -> Out/1
  Outlier-failure/1 -> Switch/1
  Mux/1 -> Gain/1
  Switch/1 -> Mux/3, Mux/1, Mux/2
  In3/1 -> Switch/2
  Pump Pressure/1 -> Switch/3
